simulink model "simulated_physical_reactor_v3"  (R2023a)
settings: Solver=FixedStepAuto  StartTime=0.0  StopTime=300  FixedStep=ts  RelTol=1e-3
values from neighbouring files (symbols this model uses):
  actionDelay = 10    [MainCode.m]
  buffer = 10    [MainCode.m]
  C0_attack_c = 0    [MainCode.m]
  C0_noise = 1    [MainCode.m]
  C0_post_attack = 0    [MainCode.m]
  C0_post_attack_val = -.25    (= -0.25)    [MainCode.m]
  Ccell0 = cell0 / v_cell    (= 15384.6153846)    [MainCode.m]
  CG0 = 185    [MainCode.m]
  CG_attack_c = 55    [MainCode.m]
  CG_attack_time = 175    [MainCode.m]
  CG_fake_failure = 0    [MainCode.m]
  CG_fake_failure_noise = 8    [MainCode.m]
  CG_increase_b = 0    [MainCode.m]
  CG_increase_rate = 2    [MainCode.m]
  cg_noGrowth = 10    [MainCode.m]
  CG_noise = 1    [MainCode.m]
  CG_post_attack = 1    [MainCode.m]
  CG_post_attack_val = .25    (= 0.25)    [MainCode.m]
  CG_ramp_attack = 1    [MainCode.m]
  CG_ramp_time = 125    [MainCode.m]
  CG_target = 50    [MainCode.m]
  CG_tolerance = .2    (= 0.2)    [MainCode.m]
  CM = 4    [MainCode.m]
  CO0 = .245    (= 0.245)    [MainCode.m]
  CO_attack_time = 80    [MainCode.m]
  CO_fake_failure = 0    [MainCode.m]
  CO_fake_failure_mean = .08    (= 0.08)    [MainCode.m]
  CO_fake_failure_noise = .005    (= 0.005)    [MainCode.m]
  CO_ramp_attack = 0    [MainCode.m]
  CO_ramp_time = 100    [MainCode.m]
  CO_tolerance = 0    [MainCode.m]
  count_thresh = 3    [MainCode.m]
  dd_counter_measure = 0    [MainCode.m]
  F_fresh_max = 25    [MainCode.m]
  F_net = F_fresh_start + F_recycle_start    (= 334.8)    [MainCode.m]
  flowrateNoiseActive = 0    [MainCode.m]
  flowrateNoiseVal = 0.5 / 100    (= 0.005)    [MainCode.m]
  fresh_attack = 0    [MainCode.m]
  fresh_attack_time = 70    [MainCode.m]
  fresh_attack_val = .1    (= 0.1)    [MainCode.m]
  freshPump_fail_time = 30    [MainCode.m]
  freshPump_failure = 0    [MainCode.m]
  freshPump_response_increases = 2    [MainCode.m]
  freshPump_response_window = 10    [MainCode.m]
  g_failure_start_t = 80    [MainCode.m]
  g_fault_wait_time = 10    [MainCode.m]
  g_flowrate_control_windowsize = 10    [MainCode.m]
  g_lownoise_val = 1.25    [MainCode.m]
  g_numpoints_fail = g_standdev_window_size+1    (= 16)    [MainCode.m]
  g_numpoints_low = 4    [MainCode.m]
  g_prob_arraylen = 15    [MainCode.m]
  g_prob_count = 6    [MainCode.m]
  g_prob_thresh = .45    (= 0.45)    [MainCode.m]
  g_standdev_window_size = 15    [MainCode.m]
  g_standev_tol = 7    [MainCode.m]
  glucose_fail_noise = 10    [MainCode.m]
  glucosesensor_failure = 0    [MainCode.m]
  lowConc_controller_onState = 1    [MainCode.m]
  mean_noise_C0 = 0    [MainCode.m]
  mean_noise_CG = 0    [MainCode.m]
  mu_max = 0.0251    [MainCode.m]
  n_size = t_window/ts    (= 2.5)    [MainCode.m]
  n_size_CG = n_size    (= 2.5)    [MainCode.m]
  o2_alpha = .20    (= 0.2)    [MainCode.m]
  o2_fail_mean = .008    (= 0.008)    [MainCode.m]
  o2_fail_noise = .005    (= 0.005)    [MainCode.m]
  o2_fail_time = 50    [MainCode.m]
  o2_fault_halfrange = .01    (= 0.01)    [MainCode.m]
  o2_fault_numpoints = 5    [MainCode.m]
  o2_lownoise_val = .0008    (= 0.0008)    [MainCode.m]
  o2_movingaverage_window = 10    [MainCode.m]
  o2_numpoints_low = 6    [MainCode.m]
  o2_prob_arraylen = 10    [MainCode.m]
  o2_prob_count = 6    [MainCode.m]
  o2_prob_thresh = .45    (= 0.45)    [MainCode.m]
  o2sensor_failure = 0    [MainCode.m]
  OCR = 2.8e-11    [MainCode.m]
  p_thresh = .4    (= 0.4)    [MainCode.m]
  rec_attack = 0    [MainCode.m]
  rec_attack_time = 50    [MainCode.m]
  rec_attack_val = 120    [MainCode.m]
  recPump_drop_val = .02    (= 0.02)    [MainCode.m]
  recPump_fail_time = 30    [MainCode.m]
  recPump_failure = 0    [MainCode.m]
  recPump_rollingavg_samples_buildup = 10    [MainCode.m]
  recPump_smallDrop_size = 0.006    [MainCode.m]
  ss_counter_measure = 0    [MainCode.m]
  stdev_noise_C0 = .002    (= 0.002)    [MainCode.m]
  stdev_noise_CG = 3.5    [MainCode.m]
  t_crit_CG = .7    (= 0.7)    [MainCode.m]
  ts = 1    [MainCode.m]
  V = 65.0    (= 65)    [MainCode.m]
  v_cell = 65    [MainCode.m]
  YGC = 155 * 10^-6    (= 0.000155)    [MainCode.m]
undefined symbols (not defined in the file or in its folder): DiscIntNeverNeededParam, recPump_numDrops_waitTime, recPump_rollingavg_numDrops
libraries: simulink x16, sldrtlib x11, dspstat3 x8, aerolibanimutils x1
(part 3 of 3)

== matlab function simulated_physical_reactor_v3/CO Attack System/MATLAB Function2 ==
  data: o2_in input; o2_out output; o2_noise input; o2_const input; isFailed input
function o2_out = o2_failure(o2_in, o2_noise, o2_const, isFailed)

if isFailed == 0
    o2_out = o2_in;
else
    o2_out = normrnd(o2_const,o2_noise);
end

== matlab function simulated_physical_reactor_v3/Attack and Fault Detection System/Steady State Detection System1/MATLAB Function4 ==
  data: input input; ABG output; n_size input
function ABG = fcn(input, n_size)

if mod(input,n_size)==0
    ABG = -1;
else
    ABG = 1;
end

== matlab function simulated_physical_reactor_v3/Simulated Reactor/MATLAB Function3 ==
  data: divide input; out output; mult input
function out = divideNotZero(divide, mult)

if divide==0
    out = 0;
else
    out = mult/divide;
end

== matlab function simulated_physical_reactor_v3/Fresh Flowrate Attack System/MATLAB Function ==
  data: flow_in input; flow_out output; attack_on input; attack_val input; attack_time input; time input
function flow_out = pumpAttack(flow_in, attack_on, attack_val, attack_time, time)

if (attack_on==1 && time>=attack_time)
    flow_out = attack_val;
else
    flow_out = flow_in;
end

== matlab function simulated_physical_reactor_v3/Recycle Flowrate Attack System/MATLAB Function ==
  data: flow_in input; flow_out output; attack_on input; attack_val input; attack_time input; time input
function flow_out = pumpAttack(flow_in, attack_on, attack_val, attack_time, time)

if (attack_on==1 && time>=attack_time)
    flow_out = attack_val;
else
    flow_out = flow_in;
end

== matlab function simulated_physical_reactor_v3/Fresh Flowrate Fault System/MATLAB Function ==
  data: in_flow input; out_flow output; fault_on input; time input; fault_time input
function out_flow = fcn(in_flow, fault_on, time, fault_time)

if (fault_on==1 && time>fault_time)
    out_flow = 0;
else
    out_flow = in_flow;
end

== matlab function simulated_physical_reactor_v3/Recycle Flowrate Fault System/MATLAB Function ==
  data: in_flow input; out_flow output; fault_on input; time input; fault_time input
function out_flow = fcn(in_flow, fault_on, time, fault_time)

if (fault_on==1 && time>fault_time)
    out_flow = 0;
else
    out_flow = in_flow;
end

== matlab function simulated_physical_reactor_v3/Glucose sensor failure/MATLAB Function ==
  data: glucose_in input; glucoseOut output; glucose_noise input; isFailed input
function glucoseOut = glucose_failure(glucose_in, glucose_noise, isFailed)

if isFailed == 0
    glucoseOut = glucose_in;
else
    r = normrnd(0,glucose_noise);
    glucoseOut = glucose_in + r;
end

== matlab function simulated_physical_reactor_v3/recycle or fresh medium1 ==
  data: fresh_flowrate input; recycled_flowrate input; CG0 input; CG_recycled input; CG_inlet output; total_flowrate output
function [CG_inlet, total_flowrate]  = isNewFluid(fresh_flowrate, recycled_flowrate, CG0, CG_recycled)

%net flowrate into reactor is fresh+recycle rates
total_flowrate = fresh_flowrate + recycled_flowrate;

%glucose concentration is sum of each fluid stream's concentrations
CG_inlet = ((fresh_flowrate*CG0) + (recycled_flowrate*CG_recycled)) / total_flowrate;
